simulink subsystem "PvtSubSys_VSM_LKA"  (R2020b)
settings: Solver=VariableStepAuto  StartTime=0.0  StopTime=10.0  RelTol=1e-3
values from neighbouring files (symbols this model uses):
  P_VSM_LKA_AbsEspInTime = 3.0    [LKA.sldd]
  P_VSM_LKA_absLongitudeAcceIn = 2.5    [LKA.sldd]
  P_VSM_LKA_absLongitudeAcceInTime = 3.0    [LKA.sldd]
  P_VSM_LKA_absLongitudeAcceOut = 3.0    [LKA.sldd]
  P_VSM_LKA_AccPedalPosnOut = 30.0    [LKA.sldd]
  P_VSM_LKA_AccPedalRateOutTime = 0.0    [LKA.sldd]
  P_VSM_LKA_AccRateIn = 30.0    [LKA.sldd]
  P_VSM_LKA_AccRateInTime = 1.5    [LKA.sldd]
  P_VSM_LKA_AccRateOut = 70.0    [LKA.sldd]
  P_VSM_LKA_BrakePressIn = 3.0    [LKA.sldd]
  P_VSM_LKA_BrakePressInTime = 1.5    [LKA.sldd]
  P_VSM_LKA_BrakePressOut = 5.0    [LKA.sldd]
  P_VSM_LKA_CurveFactor = 1.0    [LKA.sldd]
  P_VSM_LKA_DriverInputTrqValueIn = 2.0    [LKA.sldd]
  P_VSM_LKA_DriverInputTrqValueInTime = 3.0    [LKA.sldd]
  P_VSM_LKA_DriverInputTrqValueOut = 2.3    [LKA.sldd]
  P_VSM_LKA_EndSwitch = 1.0    [LKA.sldd]
  P_VSM_LKA_LaneChangeOffset = 0.11    [LKA.sldd]
  P_VSM_LKA_LaneCurveIn = 0.005    [LKA.sldd]
  P_VSM_LKA_LaneCurveOut = 0.006    [LKA.sldd]
  P_VSM_LKA_LateralAcceIn = 3.0    [LKA.sldd]
  P_VSM_LKA_LateralAcceInTime = 3.0    [LKA.sldd]
  P_VSM_LKA_LateralAcceOut = 3.5    [LKA.sldd]
  P_VSM_LKA_LongitudeAcceIn = 3.0    [LKA.sldd]
  P_VSM_LKA_LongitudeAcceOut = 3.5    [LKA.sldd]
  P_VSM_LKA_OverrideInTime = 1.5    [LKA.sldd]
  P_VSM_LKA_OverrideTime = 0.3    [LKA.sldd]
  P_VSM_LKA_OverrideValue = 1.2    [LKA.sldd]
  P_VSM_LKA_State_Absesp_enable = 1.0    [LKA.sldd]
  P_VSM_LKA_State_Accpedalrate_enable = 1.0    [LKA.sldd]
  P_VSM_LKA_State_Breakpressure_enable = 1.0    [LKA.sldd]
  P_VSM_LKA_State_DriverInputTrqValue_enable = 1.0    [LKA.sldd]
  P_VSM_LKA_State_Eps_enable = 1.0    [LKA.sldd]
  P_VSM_LKA_State_ESSSts_enable = 1.0    [LKA.sldd]
  P_VSM_LKA_State_Failsafe_enable = 1.0    [LKA.sldd]
  P_VSM_LKA_State_GEAR_enable = 1.0    [LKA.sldd]
  P_VSM_LKA_State_Handson_enable = 1.0    [LKA.sldd]
  P_VSM_LKA_State_Headingangle_enable = 1.0    [LKA.sldd]
  P_VSM_LKA_State_Lane_enable = 1.0    [LKA.sldd]
  P_VSM_LKA_State_LaneChange_enable = 1.0    [LKA.sldd]
  P_VSM_LKA_State_Lanecurve_enable = 1.0    [LKA.sldd]
  P_VSM_LKA_State_LateralAcce_enable = 1.0    [LKA.sldd]
  P_VSM_LKA_State_LongitudeAcc_enable = 1.0    [LKA.sldd]
  P_VSM_LKA_State_Overide_enable = 1.0    [LKA.sldd]
  P_VSM_LKA_State_Param_AngleOffset = 0.15    [LKA.sldd]
  P_VSM_LKA_State_Param_InterventionZoneIn = 0.4    [LKA.sldd]
  P_VSM_LKA_State_Param_InterventionZoneOut = -0.65    [LKA.sldd]
  P_VSM_LKA_State_Param_LaneCurve : value not decoded    [LKA.sldd]
  P_VSM_LKA_State_Param_LaneCurve_Offset : value not decoded    [LKA.sldd]
  P_VSM_LKA_State_Param_LaneWidth_Offset : value not decoded    [LKA.sldd]
  P_VSM_LKA_State_Param_OutOffset = 0.2    [LKA.sldd]
  P_VSM_LKA_State_Param_REInterventionZoneIn = 0.55    [LKA.sldd]
  P_VSM_LKA_State_Param_Sensitive_Offset : value not decoded    [LKA.sldd]
  P_VSM_LKA_State_SteerWheelAngle_enable = 1.0    [LKA.sldd]
  P_VSM_LKA_State_SteerWheelSpd_enable = 1.0    [LKA.sldd]
  P_VSM_LKA_State_TJASts_enable = 1.0    [LKA.sldd]
  P_VSM_LKA_State_TurnLight_enable = 1.0    [LKA.sldd]
  P_VSM_LKA_State_Vehspeed_enable = 1.0    [LKA.sldd]
  P_VSM_LKA_State_Yawsup_enable = 1.0    [LKA.sldd]
  P_VSM_LKA_SteerWheelAngleIn = 70.0    [LKA.sldd]
  P_VSM_LKA_SteerWheelAngleInTime = 3.0    [LKA.sldd]
  P_VSM_LKA_SteerWheelAngleOut = 90.0    [LKA.sldd]
  P_VSM_LKA_SteerWheelSpdIn = 150.0    [LKA.sldd]
  P_VSM_LKA_SteerWheelSpdInTime = 3.0    [LKA.sldd]
  P_VSM_LKA_SteerWheelSpdOut = 200.0    [LKA.sldd]
  P_VSM_LKA_TurnLightInTime = 3.0    [LKA.sldd]
  P_VSM_LKA_Warnarea1 = -0.55    [LKA.sldd]
  P_VSM_LKA_Warnarea2 = -0.35    [LKA.sldd]
  P_VSM_LKA_WarnInTime = 2.0    [LKA.sldd]
  P_VSM_LKA_WhelDy = 2.0    [LKA.sldd]
  P_VSM_LKA_YawRateIn = 0.2    [LKA.sldd]
  P_VSM_LKA_YawRateInTime = 1.0    [LKA.sldd]
  P_VSM_LKA_YawRateOut = 0.25    [LKA.sldd]
undefined symbols (not defined in the file or in its folder): P_VSM_LKA_AddOffset, P_VSM_LSMC_SampleTime, STATE
libraries: simulink x162
(part 3 of 5)

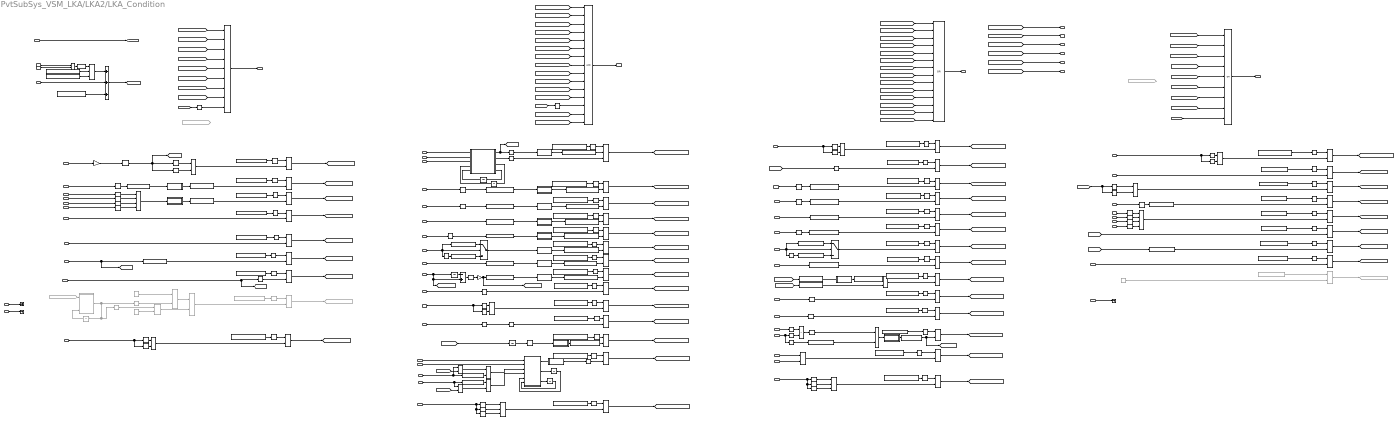
== system PvtSubSys_VSM_LKA/LKA2/LKA_Condition ==
  note: 2,3=wrong
      | 0=inactive
      | 1=active
  note: 2,3=wrong
  note: 0x0:Current gear "N" or "P"
      | 0x1:Current gear "1"
      | 0x2:Current gear "2"
      | 0x3:Current gear "3"
      | 0x4:Current gear "4"
      | 0x5:Current gear "5"
      | 0x6:Current gear "6"
      | 0x7:Current gear "7"
      | 0x8:Current gear "R"
      | 0x9-0xF:Reserved
  note: 系统当前Selected(Idle)状态非由驾驶员脱手导致
      | ∥由驾驶员脱手导致selected状态需handson
  HWAActive : Inport
  canABSVehicleSpd : Inport  Port=2
  canABMVehDynYawRate2 : Inport  Port=3
  canESPVDCActive : Inport  Port=4
  canESPPTCActive : Inport  Port=5
  canESPBTCActive : Inport  Port=6
  canABSABSActive : Inport  Port=7
  TJASts : Inport  Port=8
  Common_Lane_in : Inport  Port=9
  Headingangle_In : Inport  Port=10
  Headingangle_Out : Inport  Port=11
  LaneCurve : Inport  Port=12
  IFC_Failsafe : Inport  Port=13
  LKA_State : Inport  Port=14
  HandsOn : Inport  Port=15
  canSASSteerWheelAngle : Inport  Port=16
  canEPSEPS_DriverInputTrqValue : Inport  Port=17
  canSASSteerWheelSpd : Inport  Port=18
  canABMLateralAcce : Inport  Port=19
  LongitudeAcce : Inport  Port=20
  canESP_MasterCylindBrakePress : Inport  Port=21
  canECMAccrPedlPosnDiagc : Inport  Port=22
  canEPSEPS_LKATrqOvlDlvdSts : Inport  Port=23
  CURRENT_GEAR : Inport  Port=24
  canBCMLeftTurnSWSts : Inport  Port=25
  canBCMRightTurnSWSts : Inport  Port=26
  Common_Lane_Out : Inport  Port=27
  Scene_LaneValid : Inport  Port=28
  HandsOffWarnLevel : Inport  Port=29
  TrqK : Inport  Port=30
  Host_LRE : Inport  Port=31
  Host_RRE : Inport  Port=32
  FLWhelDy : Inport  Port=33
  FRWhelDy : Inport  Port=34
  ESSSts : Inport  Port=35
  LKA_Offset : Inport  Port=36
  LeftChange : Inport  Port=37
  RightChange : Inport  Port=38
  Abs{1,3..5,9..10,12..13,17..20} (12 alike) : Abs
  Add : Sum  Inputs=-+
  Add3 : Sum  Inputs=+++
  Bias1 : Bias  Bias=1.3
  CURRENT_GEAR1 : InportShadow  Port=24
  Compare To Constant : simulink/Logic and Bit Operations/Compare To Constant  relop=~=  const=3.0  OutDataTypeStr=boolean
  Compare To Constant1 : simulink/Logic and Bit Operations/Compare To Constant  relop=>  const=P_VSM_LKA_SteerWheelAngleInTime  OutDataTypeStr=boolean
  Compare To Constant10 : simulink/Logic and Bit Operations/Compare To Constant  relop=~=  const=5  OutDataTypeStr=boolean
  Compare To Constant11 : simulink/Logic and Bit Operations/Compare To Constant  relop===  const=5  OutDataTypeStr=boolean
  Compare To Constant{4,12,20,24,41,168..169,172,175..178,181..183,185,210,213..221,232} (27 alike) : simulink/Logic and Bit Operations/Compare To Constant  relop===  const=1  OutDataTypeStr=boolean
  Compare To Constant{2,5..6,8,17,26,31,55,81,122,125,128..129,147..148,154..155,159,164,166,189..190,192..196,199,204,207..208} (31 alike) : simulink/Logic and Bit Operations/Compare To Constant  relop===  const=0  OutDataTypeStr=boolean
  Compare To Constant123 : simulink/Logic and Bit Operations/Compare To Constant  relop=>  const=60  OutDataTypeStr=boolean
  Compare To Constant126 : simulink/Logic and Bit Operations/Compare To Constant  relop=<  const=150  OutDataTypeStr=boolean
  Compare To Constant127 : simulink/Logic and Bit Operations/Compare To Constant  Commented=on  relop===  const=0  OutDataTypeStr=boolean
  Compare To Constant13 : simulink/Logic and Bit Operations/Compare To Constant  relop=<  const=P_VSM_LKA_WhelDy  OutDataTypeStr=boolean
  Compare To Constant134 : simulink/Logic and Bit Operations/Compare To Constant  relop=>  const=P_VSM_LKA_AbsEspInTime  OutDataTypeStr=boolean
  Compare To Constant14 : simulink/Logic and Bit Operations/Compare To Constant  relop=<  const=P_VSM_LKA_WhelDy  OutDataTypeStr=boolean
  Compare To Constant15 : simulink/Logic and Bit Operations/Compare To Constant  relop===  const=4  OutDataTypeStr=boolean
  Compare To Constant150 : simulink/Logic and Bit Operations/Compare To Constant  relop=<  const=P_VSM_LKA_YawRateIn  OutDataTypeStr=boolean
  Compare To Constant153 : simulink/Logic and Bit Operations/Compare To Constant  relop=>  const=P_VSM_LKA_YawRateInTime  OutDataTypeStr=boolean
  Compare To Constant158 : simulink/Logic and Bit Operations/Compare To Constant  relop=<  const=P_VSM_LKA_LaneCurveIn  OutDataTypeStr=boolean
  Compare To Constant16 : simulink/Logic and Bit Operations/Compare To Constant  relop=~=  const=5  OutDataTypeStr=boolean
  Compare To Constant160 : simulink/Logic and Bit Operations/Compare To Constant  Commented=on  relop===  const=1  OutDataTypeStr=boolean
  Compare To Constant165 : simulink/Logic and Bit Operations/Compare To Constant  Commented=on  relop===  const=1  OutDataTypeStr=boolean
  Compare To Constant167 : simulink/Logic and Bit Operations/Compare To Constant  Commented=on  relop===  const=0  OutDataTypeStr=boolean
  Compare To Constant170 : simulink/Logic and Bit Operations/Compare To Constant  relop=<  const=55  OutDataTypeStr=boolean
  Compare To Constant171 : simulink/Logic and Bit Operations/Compare To Constant  relop=>  const=155  OutDataTypeStr=boolean
  Compare To Constant173 : simulink/Logic and Bit Operations/Compare To Constant  relop=>  const=P_VSM_LKA_YawRateOut  OutDataTypeStr=boolean
  Compare To Constant18 : simulink/Logic and Bit Operations/Compare To Constant  relop=~=  const=4  OutDataTypeStr=boolean
  Compare To Constant186 : simulink/Logic and Bit Operations/Compare To Constant  Commented=on  relop===  const=5  OutDataTypeStr=boolean
  Compare To Constant188 : simulink/Logic and Bit Operations/Compare To Constant  relop=>  const=P_VSM_LKA_LaneCurveOut  OutDataTypeStr=boolean
  Compare To Constant19 : simulink/Logic and Bit Operations/Compare To Constant  relop===  const=5  OutDataTypeStr=boolean
  Compare To Constant191 : simulink/Logic and Bit Operations/Compare To Constant  relop=<  const=P_VSM_LKA_LateralAcceIn  OutDataTypeStr=boolean
  Compare To Constant197 : simulink/Logic and Bit Operations/Compare To Constant  relop=<  const=P_VSM_LKA_BrakePressIn  OutDataTypeStr=boolean
  Compare To Constant198 : simulink/Logic and Bit Operations/Compare To Constant  relop===  const=8  OutDataTypeStr=boolean
  Compare To Constant200 : simulink/Logic and Bit Operations/Compare To Constant  relop=<  const=P_VSM_LKA_SteerWheelAngleIn  OutDataTypeStr=boolean
  Compare To Constant201 : simulink/Logic and Bit Operations/Compare To Constant  relop=<  const=2  OutDataTypeStr=boolean
  Compare To Constant202 : simulink/Logic and Bit Operations/Compare To Constant  relop=<  const=P_VSM_LKA_DriverInputTrqValueIn  OutDataTypeStr=boolean
  Compare To Constant203 : simulink/Logic and Bit Operations/Compare To Constant  relop=<  const=P_VSM_LKA_SteerWheelSpdIn  OutDataTypeStr=boolean
  Compare To Constant205 : simulink/Logic and Bit Operations/Compare To Constant  relop=<  const=P_VSM_LKA_LongitudeAcceIn  OutDataTypeStr=boolean
  Compare To Constant206 : simulink/Logic and Bit Operations/Compare To Constant  relop=<  const=P_VSM_LKA_absLongitudeAcceIn  OutDataTypeStr=boolean
  Compare To Constant209 : simulink/Logic and Bit Operations/Compare To Constant  relop=<  const=P_VSM_LKA_AccRateIn  OutDataTypeStr=boolean
  Compare To Constant21 : simulink/Logic and Bit Operations/Compare To Constant  relop===  const=4  OutDataTypeStr=boolean
  Compare To Constant211 : simulink/Logic and Bit Operations/Compare To Constant  relop=>  const=P_VSM_LKA_AccRateInTime  OutDataTypeStr=boolean
  Compare To Constant212 : simulink/Logic and Bit Operations/Compare To Constant  relop=>  const=P_VSM_LKA_TurnLightInTime  OutDataTypeStr=boolean
  Compare To Constant22 : simulink/Logic and Bit Operations/Compare To Constant  relop=~=  const=6  OutDataTypeStr=boolean
  Compare To Constant222 : simulink/Logic and Bit Operations/Compare To Constant  relop===  const=8  OutDataTypeStr=boolean
  Compare To Constant223 : simulink/Logic and Bit Operations/Compare To Constant  relop=>  const=P_VSM_LKA_SteerWheelAngleOut  OutDataTypeStr=boolean
  Compare To Constant225 : simulink/Logic and Bit Operations/Compare To Constant  relop=>  const=P_VSM_LKA_DriverInputTrqValueOut  OutDataTypeStr=boolean
  Compare To Constant226 : simulink/Logic and Bit Operations/Compare To Constant  relop=>  const=P_VSM_LKA_DriverInputTrqValueInTime  OutDataTypeStr=boolean
  Compare To Constant227 : simulink/Logic and Bit Operations/Compare To Constant  relop=>  const=P_VSM_LKA_SteerWheelSpdOut  OutDataTypeStr=boolean
  Compare To Constant228 : simulink/Logic and Bit Operations/Compare To Constant  relop=>  const=P_VSM_LKA_SteerWheelSpdInTime  OutDataTypeStr=boolean
  Compare To Constant229 : simulink/Logic and Bit Operations/Compare To Constant  relop=>  const=P_VSM_LKA_LateralAcceOut  OutDataTypeStr=boolean
  Compare To Constant23 : simulink/Logic and Bit Operations/Compare To Constant  relop=~=  const=9  OutDataTypeStr=boolean
  Compare To Constant230 : simulink/Logic and Bit Operations/Compare To Constant  relop=>  const=P_VSM_LKA_LongitudeAcceOut  OutDataTypeStr=boolean
  Compare To Constant231 : simulink/Logic and Bit Operations/Compare To Constant  relop=>  const=P_VSM_LKA_absLongitudeAcceOut  OutDataTypeStr=boolean
  Compare To Constant233 : simulink/Logic and Bit Operations/Compare To Constant  relop=>  const=P_VSM_LKA_BrakePressOut  OutDataTypeStr=boolean
  Compare To Constant234 : simulink/Logic and Bit Operations/Compare To Constant  relop=>  const=P_VSM_LKA_AccRateOut  OutDataTypeStr=boolean
  Compare To Constant235 : simulink/Logic and Bit Operations/Compare To Constant  relop=>  const=1  OutDataTypeStr=boolean
  Compare To Constant236 : simulink/Logic and Bit Operations/Compare To Constant  relop=>  const=P_VSM_LKA_BrakePressInTime  OutDataTypeStr=boolean
  Compare To Constant237 : simulink/Logic and Bit Operations/Compare To Constant  relop=>  const=P_VSM_LKA_absLongitudeAcceInTime  OutDataTypeStr=boolean
  Compare To Constant238 : simulink/Logic and Bit Operations/Compare To Constant  relop=>  const=P_VSM_LKA_LateralAcceInTime  OutDataTypeStr=boolean
  Compare To Constant25 : simulink/Logic and Bit Operations/Compare To Constant  relop=>  const=P_VSM_LKA_OverrideInTime  OutDataTypeStr=boolean
  Compare To Constant27 : simulink/Logic and Bit Operations/Compare To Constant  relop=>  const=P_VSM_LKA_AccPedalPosnOut  OutDataTypeStr=boolean
  Compare To Constant28 : simulink/Logic and Bit Operations/Compare To Constant  relop===  const=3.0  OutDataTypeStr=boolean
  Compare To Constant29 : simulink/Logic and Bit Operations/Compare To Constant  relop===  const=6  OutDataTypeStr=boolean
  Compare To Constant3 : simulink/Logic and Bit Operations/Compare To Constant  Commented=on  relop===  const=1  OutDataTypeStr=boolean
  Compare To Constant30 : simulink/Logic and Bit Operations/Compare To Constant  relop===  const=9  OutDataTypeStr=boolean
  Compare To Constant33 : simulink/Logic and Bit Operations/Compare To Constant  relop=>  const=P_VSM_LKA_AccPedalRateOutTime  OutDataTypeStr=boolean
  Compare To Constant49 : simulink/Logic and Bit Operations/Compare To Constant  relop=>  const=0.5  OutDataTypeStr=boolean
  Compare To Constant54 : simulink/Logic and Bit Operations/Compare To Constant  relop=<  const=0  OutDataTypeStr=boolean
  Compare To Constant56 : simulink/Logic and Bit Operations/Compare To Constant  relop=>  const=P_VSM_LKA_OverrideValue  OutDataTypeStr=boolean
  Compare To Constant7 : simulink/Logic and Bit Operations/Compare To Constant  relop=>  const=P_VSM_LKA_OverrideTime  OutDataTypeStr=boolean
  Compare To Constant9 : simulink/Logic and Bit Operations/Compare To Constant  relop=~=  const=4  OutDataTypeStr=boolean
  Constant1 : Constant  Value=P_VSM_LKA_LaneChangeOffset
  Constant2 : Constant  Value=P_VSM_LKA_State_Param_REInterventionZoneIn
  Constant3 : Constant  Value=P_VSM_LKA_State_Param_InterventionZoneIn
  Data Type Conversion : DataTypeConversion
  ESSSts1 : InportShadow  Port=35
  ESSSts2 : InportShadow  Port=35
  ESSSts3 : InportShadow  Port=35
  From10 : From  Commented=on  GotoTag=Con_Handson_Idle2Ready
  From105 : From  Commented=on  GotoTag=Con_HandOff_Ready2Idle
  From96 : From  Commented=on  GotoTag=Con_HandOff_Ready2Idle
  Gain : Gain  Gain=50
  Gain1 : Gain  Gain=1.03
  Goto70 : Goto  Commented=on  GotoTag=Con_Handson_Idle2Ready
  Goto83 : Goto  Commented=on  GotoTag=Con_HandOff_Ready2Idle
  LeftChange1 : InportShadow  Port=37
  Logical Operator{,1,3,9..10,13,15,18..19,77,95..96,103..105,108..109,113,125..130,132..134} (27 alike) : Logic  Operator=OR  AllPortsSameDT=off  OutDataTypeStr=boolean
  Logical Operator101 : Logic  Operator=NOT  AllPortsSameDT=off  OutDataTypeStr=boolean
  Logical Operator102 : Logic  Commented=on  AllPortsSameDT=off  OutDataTypeStr=boolean
  Logical Operator106 : Logic  Commented=on  Operator=OR  AllPortsSameDT=off  OutDataTypeStr=boolean
  Logical Operator107 : Logic  Commented=on  Operator=OR  AllPortsSameDT=off  OutDataTypeStr=boolean
  Logical Operator{4..8,11..12,16,20,47,98,112,114..115,117..120,137..146} (28 alike) : Logic  AllPortsSameDT=off  OutDataTypeStr=boolean
  Logical Operator110 : Logic  Operator=OR  Inputs=9  AllPortsSameDT=off  OutDataTypeStr=boolean
  Logical Operator116 : Logic  Operator=OR  Inputs=4  AllPortsSameDT=off  OutDataTypeStr=boolean
  Logical Operator121 : Logic  Commented=on  AllPortsSameDT=off  OutDataTypeStr=boolean
  Logical Operator123 : Logic  Inputs=15  AllPortsSameDT=off  OutDataTypeStr=boolean
  Logical Operator124 : Logic  Operator=OR  Inputs=3  AllPortsSameDT=off  OutDataTypeStr=boolean
  Logical Operator131 : Logic  Operator=NOT  AllPortsSameDT=off  OutDataTypeStr=boolean
  Logical Operator135 : Logic  Operator=OR  Inputs=14  AllPortsSameDT=off  OutDataTypeStr=boolean
  Logical Operator14 : Logic  Inputs=3  AllPortsSameDT=off  OutDataTypeStr=boolean
  Logical Operator17 : Logic  Operator=OR  Inputs=3  AllPortsSameDT=off  OutDataTypeStr=boolean
  Logical Operator2 : Logic  Commented=on  AllPortsSameDT=off  OutDataTypeStr=boolean
  Logical Operator42 : Logic  Inputs=9  AllPortsSameDT=off  OutDataTypeStr=boolean
  Logical Operator99 : Logic  Inputs=4  AllPortsSameDT=off  OutDataTypeStr=boolean
  LongitudeAcce1 : InportShadow  Port=20
  MATLAB Function : MATLAB Function  TreatAsAtomicUnit=on
  MATLAB Function1 : MATLAB Function  Commented=on  TreatAsAtomicUnit=on
  Multiport Switch : MultiPortSwitch  Inputs=2  DiagnosticForDefault=None
  Product : Product
  Relational Operator : RelationalOperator  Operator=>  OutDataTypeStr=boolean  RndMeth=Simplest
  Relational Operator1 : RelationalOperator  Operator=>  OutDataTypeStr=boolean  RndMeth=Simplest
  RightChange1 : InportShadow  Port=38
  Sign : Signum
  Sign1 : Signum
  State_TurnLight2 : MATLAB Function  TreatAsAtomicUnit=on
  Subsystem1 : Subsystem  mask{Ts=P_VSM_LSMC_SampleTime, Max=10}
      mask prompts: Ts "Sample Time:"; Max "Max Limit:"
      mask Display:
      | Ts=get_param(gcb,'Ts');
      | Max=get_param(gcb,'Max');
      | disp(['Ts:' Ts '\n' 'Max:' Max ]);
  Subsystem10 : Subsystem  mask{Ts=P_VSM_LSMC_SampleTime, Max=10}
      mask prompts: Ts "Sample Time:"; Max "Max Limit:"
      mask Display:
      | Ts=get_param(gcb,'Ts');
      | Max=get_param(gcb,'Max');
      | disp(['Ts:' Ts '\n' 'Max:' Max ]);
  Subsystem12 : Subsystem  mask{Ts=P_VSM_LSMC_SampleTime, Max=10}
      mask prompts: Ts "Sample Time:"; Max "Max Limit:"
      mask Display:
      | Ts=get_param(gcb,'Ts');
      | Max=get_param(gcb,'Max');
      | disp(['Ts:' Ts '\n' 'Max:' Max ]);
  Subsystem13 : Subsystem  mask{Ts=P_VSM_LSMC_SampleTime, Max=10}
      mask prompts: Ts "Sample Time:"; Max "Max Limit:"
      mask Display:
      | Ts=get_param(gcb,'Ts');
      | Max=get_param(gcb,'Max');
      | disp(['Ts:' Ts '\n' 'Max:' Max ]);
  Subsystem15 : Subsystem  mask{Ts=P_VSM_LSMC_SampleTime, Max=10}
      mask prompts: Ts "Sample Time:"; Max "Max Limit:"
      mask Display:
      | Ts=get_param(gcb,'Ts');
      | Max=get_param(gcb,'Max');
      | disp(['Ts:' Ts '\n' 'Max:' Max ]);
  Subsystem18 : Subsystem  mask{Ts=P_VSM_LSMC_SampleTime, Max=10}
      mask prompts: Ts "Sample Time:"; Max "Max Limit:"
      mask Display:
      | Ts=get_param(gcb,'Ts');
      | Max=get_param(gcb,'Max');
      | disp(['Ts:' Ts '\n' 'Max:' Max ]);
  Subsystem2 : Subsystem  mask{Ts=P_VSM_LSMC_SampleTime, Max=10}
      mask prompts: Ts "Sample Time:"; Max "Max Limit:"
      mask Display:
      | Ts=get_param(gcb,'Ts');
      | Max=get_param(gcb,'Max');
      | disp(['Ts:' Ts '\n' 'Max:' Max ]);
  Subsystem3 : Subsystem  mask{Ts=P_VSM_LSMC_SampleTime, Max=10}
      mask prompts: Ts "Sample Time:"; Max "Max Limit:"
      mask Display:
      | Ts=get_param(gcb,'Ts');
      | Max=get_param(gcb,'Max');
      | disp(['Ts:' Ts '\n' 'Max:' Max ]);
  Subsystem4 : Subsystem  mask{Ts=P_VSM_LSMC_SampleTime, Max=10}
      mask prompts: Ts "Sample Time:"; Max "Max Limit:"
      mask Display:
      | Ts=get_param(gcb,'Ts');
      | Max=get_param(gcb,'Max');
      | disp(['Ts:' Ts '\n' 'Max:' Max ]);
  Subsystem5 : Subsystem  mask{Ts=P_VSM_LSMC_SampleTime, Max=10}
      mask prompts: Ts "Sample Time:"; Max "Max Limit:"
      mask Display:
      | Ts=get_param(gcb,'Ts');
      | Max=get_param(gcb,'Max');
      | disp(['Ts:' Ts '\n' 'Max:' Max ]);
  Subsystem6 : Subsystem  mask{Ts=P_VSM_LSMC_SampleTime, Max=10}
      mask prompts: Ts "Sample Time:"; Max "Max Limit:"
      mask Display:
      | Ts=get_param(gcb,'Ts');
      | Max=get_param(gcb,'Max');
      | disp(['Ts:' Ts '\n' 'Max:' Max ]);
  Subsystem7 : Subsystem  mask{Ts=P_VSM_LSMC_SampleTime, Max=10}
      mask prompts: Ts "Sample Time:"; Max "Max Limit:"
      mask Display:
      | Ts=get_param(gcb,'Ts');
      | Max=get_param(gcb,'Max');
      | disp(['Ts:' Ts '\n' 'Max:' Max ]);
  Subsystem8 : Subsystem  mask{Ts=P_VSM_LSMC_SampleTime, Max=10}
      mask prompts: Ts "Sample Time:"; Max "Max Limit:"
      mask Display:
      | Ts=get_param(gcb,'Ts');
      | Max=get_param(gcb,'Max');
      | disp(['Ts:' Ts '\n' 'Max:' Max ]);
  Subsystem9 : Subsystem  mask{Ts=P_VSM_LSMC_SampleTime, Max=10}
      mask prompts: Ts "Sample Time:"; Max "Max Limit:"
      mask Display:
      | Ts=get_param(gcb,'Ts');
      | Max=get_param(gcb,'Max');
      | disp(['Ts:' Ts '\n' 'Max:' Max ]);
  Switch1 : Switch  Criteria=u2 > Threshold
  Switch3 : Switch  Criteria=u2 > Threshold
  TJASts1 : InportShadow  Port=8
  Terminator : Terminator
  Terminator1 : Terminator
  Terminator2 : Terminator
  Unit Delay{,1..5} (6 alike) : UnitDelay  SampleTime=-1  HasFrameUpgradeWarning=on
  Unit Delay7 : UnitDelay  Commented=on  SampleTime=-1  HasFrameUpgradeWarning=on
  canABMLateralAcce1 : InportShadow  Port=19
  canABMVehDynYawRate : InportShadow  Port=3
  canABSABSActive1 : InportShadow  Port=7
  canEPSEPS_DriverInputTrqValue1 : InportShadow  Port=17
  canEPSEPS_DriverInputTrqValue2 : InportShadow  Port=17
  canEPSEPS_LKATrqOvlDlvdSts1 : InportShadow  Port=23
  canESPBTCActive1 : InportShadow  Port=6
  canESPPTCActive1 : InportShadow  Port=5
  canESPVDCActive1 : InportShadow  Port=4
  canESP_MasterCylindBrakePress1 : InportShadow  Port=21
  canSASSteerWheelAngle1 : InportShadow  Port=16
  canSASSteerWheelSpd1 : InportShadow  Port=18
  param_1 : Constant  Value=P_VSM_LKA_State_Yawsup_enable
  param_10 : Constant  Value=P_VSM_LKA_State_LateralAcce_enable
  param_11 : Constant  Value=P_VSM_LKA_State_LongitudeAcc_enable
  param_12 : Constant  Value=P_VSM_LKA_State_TurnLight_enable
  param_13 : Constant  Value=P_VSM_LKA_State_Breakpressure_enable
  param_14 : Constant  Value=P_VSM_LKA_State_Accpedalrate_enable
  param_15 : Constant  Value=P_VSM_LKA_State_Overide_enable
  param_16 : Constant  Value=P_VSM_LKA_State_Eps_enable
  param_17 : Constant  Value=P_VSM_LKA_State_GEAR_enable
  param_18 : Constant  Value=P_VSM_LKA_State_Overide_enable
  param_19 : Constant  Value=P_VSM_LKA_State_LaneChange_enable
  param_2 : Constant  Value=P_VSM_LKA_State_Absesp_enable
  param_{20..23} (4 alike) : Constant  Value=P_VSM_LKA_State_ESSSts_enable
  param_24 : Constant  Value=P_VSM_LKA_State_TJASts_enable
  param_25 : Constant  Value=P_VSM_LKA_State_TJASts_enable
  param_3 : Constant  Value=P_VSM_LKA_State_Lane_enable
  param_4 : Constant  Value=P_VSM_LKA_State_Headingangle_enable
  param_5 : Constant  Value=P_VSM_LKA_State_SteerWheelAngle_enable
  param_55 : Constant  Value=P_VSM_LKA_State_Vehspeed_enable
  param_6 : Constant  Value=P_VSM_LKA_State_Failsafe_enable
  param_60 : Constant  Commented=on  Value=P_VSM_LKA_State_Handson_enable
  param_61 : Constant  Value=P_VSM_LKA_State_Lanecurve_enable
  param_63 : Constant  Value=P_VSM_LKA_State_Lane_enable
  param_64 : Constant  Value=P_VSM_LKA_State_Vehspeed_enable
  param_65 : Constant  Value=P_VSM_LKA_State_Yawsup_enable
  param_66 : Constant  Value=P_VSM_LKA_State_Absesp_enable
  param_67 : Constant  Value=P_VSM_LKA_State_Failsafe_enable
  param_68 : Constant  Value=P_VSM_LKA_State_Lanecurve_enable
  param_69 : Constant  Value=P_VSM_LKA_State_Headingangle_enable
  param_7 : Constant  Value=P_VSM_LKA_State_TurnLight_enable
  param_70 : Constant  Commented=on  Value=P_VSM_LKA_State_Handson_enable
  param_72 : Constant  Value=P_VSM_LKA_State_DriverInputTrqValue_enable
  param_8 : Constant  Value=P_VSM_LKA_State_LaneChange_enable
  param_81 : Constant  Value=P_VSM_LKA_State_Eps_enable
  param_82 : Constant  Value=P_VSM_LKA_State_Accpedalrate_enable
  param_84 : Constant  Value=P_VSM_LKA_State_SteerWheelAngle_enable
  param_85 : Constant  Value=P_VSM_LKA_State_DriverInputTrqValue_enable
  param_86 : Constant  Value=P_VSM_LKA_State_SteerWheelSpd_enable
  param_87 : Constant  Value=P_VSM_LKA_State_LateralAcce_enable
  param_88 : Constant  Value=P_VSM_LKA_State_LongitudeAcc_enable
  param_89 : Constant  Value=P_VSM_LKA_State_Breakpressure_enable
  param_9 : Constant  Value=P_VSM_LKA_State_SteerWheelSpd_enable
  param_90 : Constant  Value=P_VSM_LKA_State_GEAR_enable
  LKA_Idle2Ready : Outport
  LKA_Ready2Active : Outport  Port=2
  LKA_Active2Ready : Outport  Port=3
  LKA_Ready2Idle_Active2Idle : Outport  Port=4
  LKA_Con_SteerWheelAngle_ LKAExit : Outport  Port=5
  LKA_Con_DriverInput_ LKAExit : Outport  Port=6
  LKA_Con_SteerWheelSpd_ LKAExit : Outport  Port=7
  LKA_Con_BrakePressure_ LKAExit : Outport  Port=8
  LKA_Con_AccPedalRate_LKAExit : Outport  Port=9
  LKA_Con_OverRide_ LKAExit : Outport  Port=10
  wires:
  Compare To Constant33/1 -> Logical Operator20/1
  Compare To Constant234/1 -> Subsystem13/1(In1)
  Subsystem13/1(Out1) -> Compare To Constant33/1
  Logical Operator20/1 -> Logical Operator139/2
  Compare To Constant27/1 -> Logical Operator20/2
  [AccPedalPosn] -> Compare To Constant27/1
  HandsOffWarnLevel/1 -> Terminator2/1
  HandsOn/1 -> Terminator1/1
  LKA_State/1 -> Terminator/1
  [Con_ESSSts_Idle2Ready] -> Logical Operator42/5
  ? -> Compare To Constant165/1
  Unit Delay7/1 -> MATLAB Function1/3(yK1)
  ? -> MATLAB Function1/2(LKASts)
  From96/1 -> MATLAB Function1/1(HandsOff_Ready2Idle)
  [Con_TJASts_Active2Ready] -> Logical Operator135/14
  TJASts1/1 -> Compare To Constant28/1, Compare To Constant30/1, Compare To Constant29/1
  Compare To Constant28/1 -> Logical Operator17/1
  Compare To Constant30/1 -> Logical Operator17/3
  Compare To Constant29/1 -> Logical Operator17/2
  Logical Operator17/1 -> Logical Operator19/2
  param_25/1 -> Compare To Constant31/1
  Logical Operator19/1 -> [Con_TJASts_Active2Ready]  "VSM_LKA_Con_TJASts_Active2Ready"
  Compare To Constant31/1 -> Logical Operator19/1
  [Con_TJASts_Ready2Active] -> Logical Operator123/15
  Compare To Constant26/1 -> Logical Operator15/1
  Logical Operator15/1 -> [Con_TJASts_Ready2Active]  "VSM_LKA_Con_TJASts_Ready2Active"
  param_24/1 -> Compare To Constant26/1
  Logical Operator14/1 -> Logical Operator15/2
  Compare To Constant22/1 -> Logical Operator14/2
  Compare To Constant23/1 -> Logical Operator14/3
  Compare To Constant/1 -> Logical Operator14/1
  TJASts/1 -> Compare To Constant/1, Compare To Constant22/1, Compare To Constant23/1
  Gain/1 -> Compare To Constant209/1, [AccPedalRate]
  Abs1/1 -> Gain/1
  Logical Operator13/1 -> Logical Operator12/2
  Compare To Constant19/1 -> Logical Operator13/2
  Compare To Constant21/1 -> Logical Operator13/1
  Compare To Constant20/1 -> Logical Operator12/1
  Logical Operator12/1 -> [Con_ESSSts_Ready2Idle]  "VSM_LKA_Con_ESSSts_Ready2Idle"
  ESSSts3/1 -> Compare To Constant21/1, Compare To Constant19/1
  param_23/1 -> Compare To Constant20/1
  param_22/1 -> Compare To Constant17/1
  ESSSts2/1 -> Compare To Constant16/1, Compare To Constant18/1
  Logical Operator10/1 -> [Con_ESSSts_Idle2Ready]  "VSM_LKA_Con_ESSSts_Idle2Ready"
  Compare To Constant17/1 -> Logical Operator10/1
  Compare To Constant18/1 -> Logical Operator11/1
  Compare To Constant16/1 -> Logical Operator11/2
  Logical Operator11/1 -> Logical Operator10/2
  [Con_ESSSts_Active2Ready] -> Logical Operator135/13
  param_21/1 -> Compare To Constant12/1
  ESSSts1/1 -> Compare To Constant11/1, Compare To Constant15/1
  Logical Operator8/1 -> [Con_ESSSts_Active2Ready]  "VSM_LKA_Con_ESSSts_Active2Ready"
  Compare To Constant12/1 -> Logical Operator8/1
  Compare To Constant15/1 -> Logical Operator9/1
  Compare To Constant11/1 -> Logical Operator9/2
  Logical Operator9/1 -> Logical Operator8/2
  [Con_ESSSts_Ready2Active] -> Logical Operator123/14
  Logical Operator4/1 -> Logical Operator1/2
  Compare To Constant10/1 -> Logical Operator4/2
  Compare To Constant9/1 -> Logical Operator4/1
  Compare To Constant8/1 -> Logical Operator1/1
  Logical Operator1/1 -> [Con_ESSSts_Ready2Active]
  ESSSts/1 -> Compare To Constant9/1, Compare To Constant10/1
  param_20/1 -> Compare To Constant8/1
  [ReactionZoneInDy] -> Relational Operator1/2
  Host_LRE/1 -> Logical Operator/1
  Add3/1 -> [ReactionZoneInDy]
  Multiport Switch/1 -> Add3/1
  Constant2/1 -> Multiport Switch/2
  LKA_Offset/1 -> Add3/2
  Logical Operator/1 -> Data Type Conversion/1
  Data Type Conversion/1 -> Multiport Switch/1
  Host_RRE/1 -> Logical Operator/2
  Constant3/1 -> Multiport Switch/3
  Constant1/1 -> Add3/3
  Relational Operator1/1 -> Logical Operator6/1
  Relational Operator/1 -> Logical Operator7/2
  Compare To Constant13/1 -> Logical Operator6/2
  Compare To Constant14/1 -> Logical Operator7/1
  [ReactionZoneInDy] -> Relational Operator/2
  FRWhelDy/1 -> Relational Operator/1, Compare To Constant14/1
  FLWhelDy/1 -> Compare To Constant13/1, Relational Operator1/1
  Logical Operator6/1 -> MATLAB Function/3(Ldy)  "LKA_Ldy"
  Logical Operator7/1 -> MATLAB Function/4(Rdy)  "LKA_Rdy"
  Compare To Constant49/1 -> Logical Operator18/2
  Subsystem10/1(Out1) -> Compare To Constant49/1
  Compare To Constant7/1 -> Logical Operator16/2, [Overide_condition]
  Subsystem15/1(Out1) -> Compare To Constant7/1
  RightChange/1 -> MATLAB Function/2(RightChangefg)
  LeftChange/1 -> MATLAB Function/1(LeftChangefg)
  MATLAB Function/1(y) -> Subsystem10/1(In1)
  MATLAB Function/3(Rfg) -> Unit Delay5/1
  Unit Delay5/1 -> MATLAB Function/6(Rfgk1)
  MATLAB Function/2(Lfg) -> Unit Delay4/1
  Unit Delay4/1 -> MATLAB Function/5(Lfgk1)
  Logical Operator3/1 -> Logical Operator5/2
  RightChange1/1 -> Logical Operator3/2
  LeftChange1/1 -> Logical Operator3/1
  [HWAActive] -> Logical Operator110/9
  Compare To Constant6/1 -> Logical Operator123/13
  [HWAActive] -> Compare To Constant6/1
  Compare To Constant5/1 -> Logical Operator42/9
  [HWAActive] -> Compare To Constant5/1
  HWAActive/1 -> [HWAActive]
  param_19/1 -> Compare To Constant2/1
  param_18/1 -> Compare To Constant81/1
  param_16/1 -> Compare To Constant192/1
  param_13/1 -> Compare To Constant194/1
  param_11/1 -> Compare To Constant193/1
  param_10/1 -> Compare To Constant208/1
  param_9/1 -> Compare To Constant207/1
  param_5/1 -> Compare To Constant196/1
  param_7/1 -> Compare To Constant190/1
  param_4/1 -> Compare To Constant147/1
  param_3/1 -> Compare To Constant122/1
  param_2/1 -> Compare To Constant166/1
  param_1/1 -> Compare To Constant164/1
  [Con_LaneChange_Ready2Active] -> Logical Operator123/12
  Compare To Constant4/1 -> Logical Operator124/3
  State_TurnLight2/2(out) -> Compare To Constant4/1
  canBCMRightTurnSWSts/1 -> State_TurnLight2/2(rightlight)
  canBCMLeftTurnSWSts/1 -> State_TurnLight2/1(leftlight)
  Scene_LaneValid/1 -> State_TurnLight2/3(lane)
  Unit Delay3/1 -> State_TurnLight2/4(leftk1)
  Unit Delay2/1 -> State_TurnLight2/5(rightk1)
  State_TurnLight2/4(right) -> Unit Delay2/1
  State_TurnLight2/3(left) -> Unit Delay3/1
  Unit Delay1/1 -> Add/1
  canECMAccrPedlPosnDiagc/1 -> Unit Delay1/1, Add/2, [AccPedalPosn]
  Add/1 -> Abs1/1
  Compare To Constant3/1 -> Logical Operator2/1
  Logical Operator2/1 -> Logical Operator106/2
  Logical Operator18/1 -> [Con_LaneChange_Ready2Active]  "VSM_LKA_Con_LaneChange_Ready2Active"
  Compare To Constant2/1 -> Logical Operator18/1
  Logical Operator5/1 -> [Con_LaneChange_Active2Ready]  "VSM_LKA_Con_LaneChange_Active2Ready"
  param_8/1 -> Compare To Constant24/1
  Compare To Constant24/1 -> Logical Operator5/1
  [Con_LaneChange_Active2Ready] -> Logical Operator135/12
  [Con_Override_Ready2Active] -> Logical Operator123/11
  Unit Delay/1 -> Compare To Constant55/1
  Compare To Constant25/1 -> Logical Operator77/2
  Compare To Constant55/1 -> Subsystem12/1(In1)
  Subsystem12/1(Out1) -> Compare To Constant25/1
  Logical Operator77/1 -> [Con_Override_Ready2Active]  "VSM_LKA_Con_Override_Ready2Active"
  Compare To Constant81/1 -> Logical Operator77/1
  [Overide_condition] -> Unit Delay/1
  canEPSEPS_DriverInputTrqValue1/1 -> Abs3/1, Sign1/1
  Sign1/1 -> Product/2
  Sign/1 -> Product/1
  Logical Operator16/1 -> [Con_OverRide_Active2Ready]  "VSM_LKA_Con_OverRide_Active2Ready"
  Logical Operator47/1 -> Subsystem15/1(In1)
  Compare To Constant41/1 -> Logical Operator16/1
  Abs3/1 -> Compare To Constant56/1
  Product/1 -> Compare To Constant54/1
  Compare To Constant56/1 -> Logical Operator47/2
  Compare To Constant54/1 -> Logical Operator47/1
  param_15/1 -> Compare To Constant41/1
  TrqK/1 -> Sign/1
  Subsystem9/1(Out1) -> Compare To Constant212/1
  Compare To Constant189/1 -> Subsystem9/1(In1)
  Compare To Constant212/1 -> Logical Operator124/2
  Subsystem8/1(Out1) -> Compare To Constant1/1
  Compare To Constant200/1 -> Subsystem8/1(In1)
  Compare To Constant1/1 -> Logical Operator125/2
  Subsystem7/1(Out1) -> Compare To Constant226/1
  Compare To Constant202/1 -> Subsystem7/1(In1)
  Compare To Constant226/1 -> Logical Operator126/2
  Subsystem5/1(Out1) -> Compare To Constant228/1
  Compare To Constant203/1 -> Subsystem5/1(In1)
  Compare To Constant228/1 -> Logical Operator127/2
  Subsystem4/1(Out1) -> Compare To Constant238/1
  Compare To Constant191/1 -> Subsystem4/1(In1)
  Compare To Constant238/1 -> Logical Operator128/2
  Subsystem3/1(Out1) -> Compare To Constant237/1
  Switch1/1 -> Subsystem3/1(In1)
  Compare To Constant237/1 -> Logical Operator130/2
  Subsystem2/1(Out1) -> Compare To Constant236/1
  Compare To Constant197/1 -> Subsystem2/1(In1)
  Compare To Constant236/1 -> Logical Operator133/2
  Subsystem1/1(Out1) -> Compare To Constant211/1
  Compare To Constant209/1 -> Subsystem1/1(In1)
  Compare To Constant211/1 -> Logical Operator134/2
  Headingangle_In/1 -> Logical Operator108/2
  canABSABSActive1/1 -> Compare To Constant176/1
  canESPBTCActive1/1 -> Compare To Constant181/1
  canESPPTCActive1/1 -> Compare To Constant178/1
  canESPVDCActive1/1 -> Compare To Constant177/1
  [Con_TurnLight_Active2Ready] -> Logical Operator135/11
  Logical Operator135/1 -> LKA_Active2Ready/1  "VSM_LKA_Active2Ready"
  [Con_TurnLight_Ready2Active] -> Logical Operator123/10
  Logical Operator123/1 -> LKA_Ready2Active/1  "VSM_LKA_Ready2Active"
  [Con_VehicleSpeed_Ready2Idle] -> Logical Operator110/8
  [Con_Lane_Ready2Idle] -> Logical Operator110/7
  Logical Operator42/1 -> LKA_Idle2Ready/1  "VSM_LKA_Idle2Ready"
  [Con_VehicleSpeed_Idle2Ready] -> Logical Operator42/8
  [Con_Lane_Idle2Ready] -> Logical Operator42/7
  Logical Operator95/1 -> [Con_Lane_Idle2Ready]  "VSM_LKA_Con_Lane_Idle2Ready"
  Compare To Constant220/1 -> Logical Operator141/1
  Compare To Constant123/1 -> Logical Operator98/1
  canABMLateralAcce1/1 -> Abs19/1
  Abs20/1 -> Compare To Constant223/1
  Logical Operator98/1 -> Logical Operator96/2
  Compare To Constant210/1 -> Logical Operator141/2
  Compare To Constant215/1 -> Logical Operator137/1
  canABMLateralAcce/1 -> Abs10/1
  Logical Operator96/1 -> [Con_VehicleSpeed_Idle2Ready]  "VSM_LKA_Con_VehicleSpeed_Idle2Ready"
  [Con_Headingangle_Ready2Idle] -> Logical Operator110/5
  [Con_LaneCurve_Idle2Ready] -> Logical Operator42/6
  Compare To Constant122/1 -> Logical Operator95/1
  Compare To Constant126/1 -> Logical Operator98/2
  param_84/1 -> Compare To Constant219/1
  Compare To Constant222/1 -> Logical Operator142/2
  Compare To Constant125/1 -> Logical Operator96/1
  [Con_AccPedalRate_Ready2Active] -> Logical Operator123/7
  param_55/1 -> Compare To Constant125/1
  Compare To Constant147/1 -> Logical Operator108/1
  Compare To Constant219/1 -> Logical Operator145/1
  Gain1/1 -> Bias1/1
  param_82/1 -> Compare To Constant213/1
  param_70/1 -> Logical Operator121/1
  Compare To Constant198/1 -> Logical Operator131/1
  Bias1/1 -> Compare To Constant123/1, Compare To Constant126/1, [speed]
  Compare To Constant221/1 -> Logical Operator142/1
  canSASSteerWheelSpd1/1 -> Compare To Constant227/1
  canSASSteerWheelSpd/1 -> Compare To Constant203/1
  canEPSEPS_LKATrqOvlDlvdSts1/1 -> Compare To Constant235/1
  [AccPedalRate] -> Compare To Constant234/1
  Compare To Constant232/1 -> Logical Operator138/1
  LongitudeAcce1/1 -> Switch3/2, Compare To Constant230/1, Abs18/1
  canSASSteerWheelAngle1/1 -> Abs20/1
  canESP_MasterCylindBrakePress1/1 -> Compare To Constant233/1
  Abs19/1 -> Compare To Constant229/1
  canEPSEPS_DriverInputTrqValue2/1 -> Abs17/1
  Compare To Constant233/1 -> Logical Operator138/2
  [Con_Failsafe_Ready2Idle] -> Logical Operator110/3
  Logical Operator145/1 -> [Con_SteerWheelAngle_Active2Ready]  "VSM_LKA_Con_SteerWheelAngle_Active2Ready"
  [Con_OverRide_Active2Ready] -> Logical Operator135/9
  [Con_YawRate_Idle2Ready] -> Logical Operator42/1
  param_89/1 -> Compare To Constant232/1
  Logical Operator143/1 -> [Con_DriverInput_Active2Ready]  "VSM_LKA_Con_DriverInput_Active2Ready"
  Logical Operator142/1 -> [Con_CURRENT_GEAR_Active2Ready]  "VSM_LKA_Con_CURRENT_GEAR_Active2Ready"
  Subsystem6/1(Out1) -> Compare To Constant153/1
  Logical Operator144/1 -> [Con_SteerWheelSpd_Active2Ready]  "VSM_LKA_Con_SteerWheelSpd_Active2Ready"
  Compare To Constant214/1 -> Logical Operator140/1
  CURRENT_GEAR1/1 -> Compare To Constant222/1
  Switch3/1 -> Logical Operator137/2
  Logical Operator138/1 -> [Con_BrakePressure_Active2Ready]  "VSM_LKA_Con_BrakePressure_Active2Ready"
  Compare To Constant231/1 -> Switch3/3
  Compare To Constant229/1 -> Logical Operator146/2
  param_86/1 -> Compare To Constant217/1
  param_90/1 -> Compare To Constant221/1
  Compare To Constant213/1 -> Logical Operator139/1
  Abs17/1 -> Compare To Constant225/1
  Compare To Constant150/1 -> Subsystem6/1(In1)
  Compare To Constant235/1 -> Logical Operator140/2
  Logical Operator146/1 -> [Con_LateralAcc_Active2Ready]  "VSM_LKA_Con_LateralAcc_Active2Ready"
  Abs13/1 -> Compare To Constant206/1
  Compare To Constant208/1 -> Logical Operator128/1
  Abs18/1 -> Compare To Constant231/1
  Logical Operator113/1 -> Logical Operator114/2
  Logical Operator137/1 -> [Con_LongitudeAcc_Active2Ready]  "VSM_LKA_Con_LongitudeAcc_Active2Ready"
  Logical Operator112/1 -> [Con_Lane_Ready2Idle]  "VSM_LKA_Con_Lane_Ready2Idle"
  Logical Operator139/1 -> [Con_AccPedalRate_Active2Ready]  "VSM_LKA_Con_AccPedalRate_Active2Ready"
  param_72/1 -> Compare To Constant204/1
  Compare To Constant223/1 -> Logical Operator145/2
  Compare To Constant230/1 -> Switch3/1
  Compare To Constant218/1 -> Logical Operator143/1
  Compare To Constant225/1 -> Logical Operator143/2
  param_87/1 -> Compare To Constant216/1
  [IFC_Failsafe] -> Logical Operator118/2
  param_88/1 -> Compare To Constant215/1
  Compare To Constant172/1 -> Logical Operator115/1
  Logical Operator140/1 -> [Con_EpsSta_Active2Ready]  "VSM_LKA_Con_EpsSta_Active2Ready"
  canABMVehDynYawRate/1 -> Abs4/1
  Compare To Constant227/1 -> Logical Operator144/2
  param_85/1 -> Compare To Constant218/1
  Compare To Constant217/1 -> Logical Operator144/1
  [Con_SteerWheelSpd_Active2Ready] -> Logical Operator135/3
  param_68/1 -> Compare To Constant183/1
  param_81/1 -> Compare To Constant214/1
  [Turnlight] -> Compare To Constant210/1
  Logical Operator114/1 -> [Con_VehicleSpeed_Ready2Idle]  "VSM_LKA_Con_VehicleSpeed_Ready2Idle"
  param_12/1 -> Compare To Constant220/1
  Compare To Constant216/1 -> Logical Operator146/1
  Logical Operator131/1 -> Logical Operator132/2
  Logical Operator141/1 -> [Con_TurnLight_Active2Ready]  "VSM_LKA_Con_TurnLight_Active2Ready"
  Compare To Constant170/1 -> Logical Operator113/1
  CURRENT_GEAR/1 -> Compare To Constant198/1
  canSASSteerWheelAngle/1 -> Abs9/1
  LongitudeAcce/1 -> Switch1/2, Compare To Constant205/1, Abs13/1
  canEPSEPS_DriverInputTrqValue/1 -> Abs12/1
  [Con_AbsEsp_Idle2Ready] -> Logical Operator42/2
  canEPSEPS_LKATrqOvlDlvdSts/1 -> Compare To Constant201/1
  canESP_MasterCylindBrakePress/1 -> Compare To Constant197/1
  Abs4/1 -> Compare To Constant150/1
  Compare To Constant175/1 -> Logical Operator117/1
  Compare To Constant176/1 -> Logical Operator116/4
  Compare To Constant177/1 -> Logical Operator116/1
  param_66/1 -> Compare To Constant175/1
  Logical Operator116/1 -> Logical Operator117/2  "absespsup"
  Common_Lane_Out/1 -> Logical Operator112/2
  Compare To Constant193/1 -> Logical Operator130/1
  canABMVehDynYawRate2/1 -> Abs5/1
  Compare To Constant169/1 -> Logical Operator114/1
  Compare To Constant181/1 -> Logical Operator116/3
  Compare To Constant178/1 -> Logical Operator116/2
  Logical Operator117/1 -> [Con_AbsEsp_Ready2Idle]  "VSM_LKA_Con_AbsEsp_Ready2Idle"
  Logical Operator109/1 -> [Con_Failsafe_Idle2Ready]  "VSM_LKA_Con_Failsafe_Idle2Ready"
  Logical Operator132/1 -> [Con_CURRENT_GEAR_Ready2Active]  "VSM_LKA_Con_CURRENT_GEAR_Ready2Active"
  Logical Operator127/1 -> [Con_SteerWheelSpd_Ready2Active]  "VSM_LKA_Con_SteerWheelSpd_Ready2Active"
  Abs12/1 -> Compare To Constant202/1
  Compare To Constant205/1 -> Switch1/1
  Logical Operator126/1 -> [Con_DriverInput_Ready2Active]  "VSM_LKA_Con_DriverInput_Ready2Active"
  param_60/1 -> Compare To Constant127/1
  Abs9/1 -> Compare To Constant200/1
  Logical Operator105/1 -> [Con_LaneCurve_Idle2Ready]  "VSM_LKA_Con_LaneCurve_Idle2Ready"
  Logical Operator125/1 -> [Con_SteerWheelAngle_Ready2Active]  "VSM_LKA_Con_SteerWheelAngle_Ready2Active"
  Compare To Constant195/1 -> Logical Operator134/1
  Logical Operator110/1 -> LKA_Ready2Idle_Active2Idle/1  "VSM_LKA_Other2Idle"
  Compare To Constant196/1 -> Logical Operator125/1
  Compare To Constant129/1 -> Logical Operator105/1
  param_14/1 -> Compare To Constant195/1
  Abs10/1 -> Compare To Constant191/1
  param_6/1 -> Compare To Constant148/1
  Compare To Constant194/1 -> Logical Operator133/1
  Logical Operator129/1 -> [Con_EpsSta_Ready2Active]  "VSM_LKA_Con_EpsSta_Ready2Active"
  Compare To Constant128/1 -> Logical Operator99/4
  Logical Operator133/1 -> [Con_BrakePressure_Ready2Active]  "VSM_LKA_Con_BrakePressure_Ready2Active"
  Compare To Constant192/1 -> Logical Operator129/1
  Compare To Constant204/1 -> Logical Operator126/1
  Logical Operator130/1 -> [Con_LongitudeAcc_Ready2Active]  "VSM_LKA_Con_LongitudeAcc_Ready2Active"
  Logical Operator120/1 -> [Con_LaneCurve_Ready2Idle]  "VSM_LKA_Con_LaneCurve_Ready2Idle"
  [Con_CURRENT_GEAR_Active2Ready] -> Logical Operator135/10
  Compare To Constant207/1 -> Logical Operator127/1
  Logical Operator134/1 -> [Con_AccPedalRate_Ready2Active]  "VSM_LKA_Con_AccPedalRate_Ready2Active"
  [Con_BrakePressure_Ready2Active] -> Logical Operator123/6
  Compare To Constant206/1 -> Switch1/3
  param_17/1 -> Compare To Constant199/1
  Logical Operator128/1 -> [Con_LateralAcc_Ready2Active]  "VSM_LKA_Con_LateralAcc_Ready2Active"
  Compare To Constant201/1 -> Logical Operator129/2
  Compare To Constant199/1 -> Logical Operator132/1
  Logical Operator119/1 -> [Con_Headingangle_Ready2Idle]  "VSM_LKA_Con_Headingangle_Ready2Idle"
  Headingangle_Out/1 -> Logical Operator119/2
  param_69/1 -> Compare To Constant185/1
  Compare To Constant164/1 -> Logical Operator103/1
  Compare To Constant190/1 -> Logical Operator124/1
  Logical Operator121/1 -> Goto83/1  "VSM_LKA_Con_HandsOff_Ready2Idle"
  Compare To Constant183/1 -> Logical Operator120/1
  Compare To Constant185/1 -> Logical Operator119/1
  Compare To Constant188/1 -> Logical Operator120/2
  [Con_BrakePressure_Active2Ready] -> Logical Operator135/6
  Abs5/1 -> Compare To Constant173/1
  State_TurnLight2/1(state) -> Compare To Constant189/1, [Turnlight]
  Compare To Constant166/1 -> Logical Operator104/1
  [LaneCurve] -> Compare To Constant188/1
  Compare To Constant186/1 -> Logical Operator121/2
  [Con_LateralAcc_Active2Ready] -> Logical Operator135/4
  [Con_LongitudeAcc_Ready2Active] -> Logical Operator123/5
  param_63/1 -> Compare To Constant168/1
  [Con_EpsSta_Ready2Active] -> Logical Operator123/8
  [Con_CURRENT_GEAR_Ready2Active] -> Logical Operator123/9
  canESPPTCActive/1 -> Compare To Constant155/1
  [Con_LateralAcc_Ready2Active] -> Logical Operator123/4
  [Con_SteerWheelSpd_Ready2Active] -> Logical Operator123/3
  [Con_ESSSts_Ready2Idle] -> Logical Operator110/6
  [Con_DriverInput_Ready2Active] -> Logical Operator123/2
  [Con_SteerWheelAngle_Ready2Active] -> Logical Operator123/1
  canABSABSActive/1 -> Compare To Constant128/1
  Logical Operator124/1 -> [Con_TurnLight_Ready2Active]  "VSM_LKA_Con_TurnLight_Ready2Active"
  [Con_Failsafe_Idle2Ready] -> Logical Operator42/4
  [Con_Headingangle_Idle2Ready] -> Logical Operator42/3
  Common_Lane_in/1 -> Logical Operator95/2
  canABSVehicleSpd/1 -> Gain1/1
  Logical Operator106/1 -> Logical Operator107/2
  Logical Operator103/1 -> [Con_YawRate_Idle2Ready]  "VSM_LKA_Con_YawRate_Idle2Ready"
  Logical Operator107/1 -> Goto70/1  "VSM_LKA_Con_Handson_Idle2Ready"
  Logical Operator108/1 -> [Con_Headingangle_Idle2Ready]  "VSM_LKA_Con_Headingangle_Idle2Ready"
  Compare To Constant127/1 -> Logical Operator107/1
  Compare To Constant148/1 -> Logical Operator109/1
  Compare To Constant159/1 -> Logical Operator99/3
  Compare To Constant155/1 -> Logical Operator99/2
  MATLAB Function1/1(y) -> Unit Delay7/1, Compare To Constant3/1, Compare To Constant167/1
  Compare To Constant154/1 -> Logical Operator99/1
  Logical Operator99/1 -> Subsystem18/1(In1)
  Logical Operator104/1 -> [Con_AbsEsp_Idle2Ready]  "VSM_LKA_Con_AbsEsp_Idle2Ready"
  Compare To Constant153/1 -> Logical Operator103/2
  Logical Operator101/1 -> Logical Operator109/2
  param_61/1 -> Compare To Constant129/1
  Compare To Constant165/1 -> Logical Operator102/1
  Compare To Constant167/1 -> Logical Operator102/2
  [Con_AbsEsp_Ready2Idle] -> Logical Operator110/2
  Logical Operator102/1 -> Logical Operator106/1
  Compare To Constant160/1 -> Logical Operator2/2
  Subsystem18/1(Out1) -> Compare To Constant134/1
  Compare To Constant134/1 -> Logical Operator104/2
  Compare To Constant158/1 -> Logical Operator105/2
  [Con_SteerWheelAngle_Active2Ready] -> Logical Operator135/1
  [Con_AccPedalRate_Active2Ready] -> Logical Operator135/7
  [Con_EpsSta_Active2Ready] -> Logical Operator135/8
  [Con_DriverInput_Active2Ready] -> Logical Operator135/2
  [Con_LongitudeAcc_Active2Ready] -> Logical Operator135/5
  Compare To Constant173/1 -> Logical Operator115/2
  [Con_YawRate_Ready2Idle] -> Logical Operator110/1
  [Con_LaneCurve_Ready2Idle] -> Logical Operator110/4
  Logical Operator118/1 -> [Con_Failsafe_Ready2Idle]  "VSM_LKA_Con_Failsafe_Ready2Idle"
  param_67/1 -> Compare To Constant182/1
  Compare To Constant182/1 -> Logical Operator118/1
  canESPVDCActive/1 -> Compare To Constant154/1
  Compare To Constant168/1 -> Logical Operator112/1
  canESPBTCActive/1 -> Compare To Constant159/1
  [speed] -> Compare To Constant171/1, Compare To Constant170/1
  param_65/1 -> Compare To Constant172/1
  Logical Operator115/1 -> [Con_YawRate_Ready2Idle]  "VSM_LKA_Con_YawRate_Ready2Idle"
  Compare To Constant171/1 -> Logical Operator113/2
  param_64/1 -> Compare To Constant169/1
  IFC_Failsafe/1 -> [IFC_Failsafe], Logical Operator101/1
  LaneCurve/1 -> Compare To Constant158/1, [LaneCurve]
  [Con_SteerWheelAngle_Active2Ready] -> LKA_Con_SteerWheelAngle_ LKAExit/1  "LKA_Con_SteerWheelAngle_ LKAExit"
  [Con_DriverInput_Active2Ready] -> LKA_Con_DriverInput_ LKAExit/1  "LKA_Con_DriverInput_ LKAExit"
  [Con_SteerWheelSpd_Active2Ready] -> LKA_Con_SteerWheelSpd_ LKAExit/1  "LKA_Con_SteerWheelSpd_ LKAExit"
  [Con_BrakePressure_Active2Ready] -> LKA_Con_BrakePressure_ LKAExit/1  "LKA_Con_BrakePressure_ LKAExit"
  [Con_AccPedalRate_Active2Ready] -> LKA_Con_AccPedalRate_LKAExit/1  "LKA_Con_AccPedalRate_LKAExit"
  [Con_OverRide_Active2Ready] -> LKA_Con_OverRide_ LKAExit/1  "LKA_Con_OverRide_ LKAExit"
  ? -> Compare To Constant160/1
